simulink model "Sim_Ex32_Quiz"  (R2017a)
settings: Solver=VariableStepAuto  StartTime=0.0  StopTime=Stop_Time  MaxStep=100e-6  RelTol=1e-3
undefined symbols (not defined in the file or in its folder): Grid, PLL
settings Model: SimulationMode=accelerator  Creator=Joonhee  LastModifiedBy=Joonhee

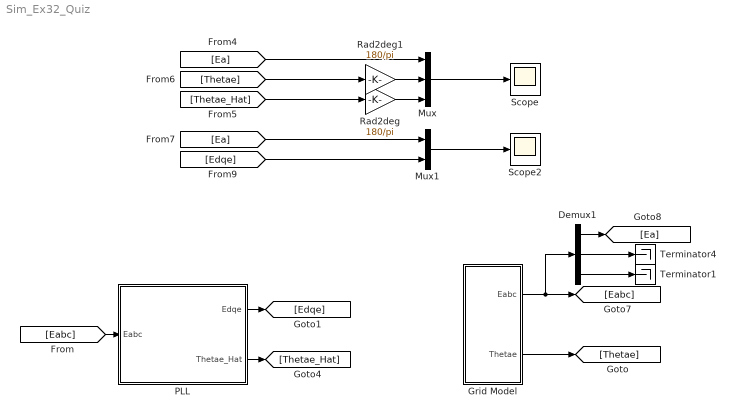
== system Sim_Ex32_Quiz ==
  Demux1 : Demux  Outputs=3
  Grid Model : Subsystem
  Mux : Mux  Inputs=3
  Mux1 : Mux  Inputs=2
  PLL : Subsystem  TreatAsAtomicUnit=on
  Rad2deg : Gain  Gain=180/pi
  Rad2deg1 : Gain  Gain=180/pi
  Scope : Scope
  Scope2 : Scope
  Terminator1 : Terminator
  Terminator4 : Terminator
  wires:
  Mux/1 -> Scope/1
  [Thetae_Hat] -> Rad2deg/1
  Rad2deg/1 -> Mux/3
  [Thetae] -> Rad2deg1/1
  Rad2deg1/1 -> Mux/2
  [Ea] -> Mux/1
  Mux1/1 -> Scope2/1
  [Ea] -> Mux1/1
  [Edqe] -> Mux1/2
  PLL/2(Thetae_Hat) -> [Thetae_Hat]
  PLL/1(Edqe) -> [Edqe]
  Demux1/1 -> [Ea]
  Demux1/2 -> Terminator4/1
  Demux1/3 -> Terminator1/1
  Grid Model/1(Eabc) -> Demux1/1, [Eabc]
  Grid Model/2(Thetae) -> [Thetae]
  [Eabc] -> PLL/1(Eabc)

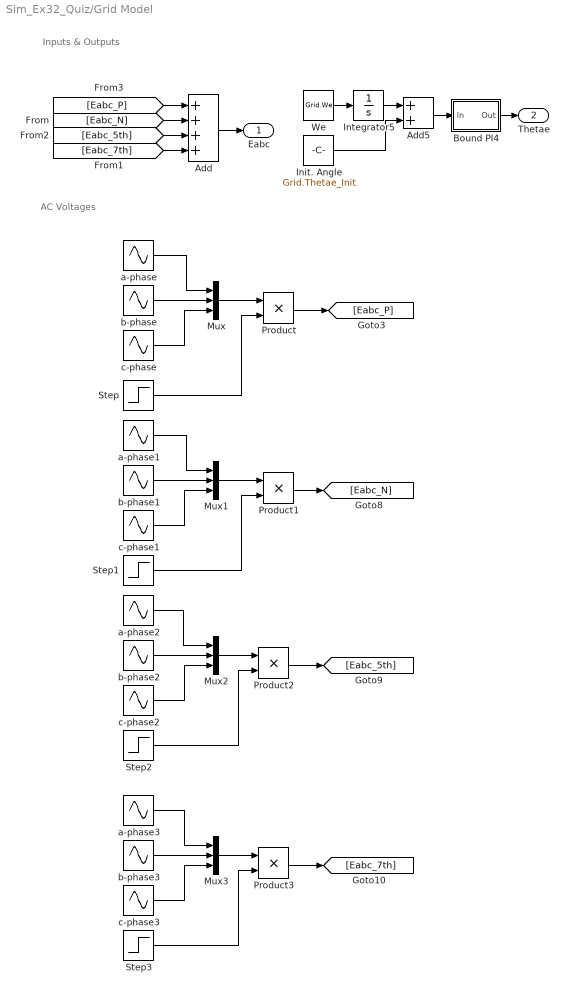
== system Sim_Ex32_Quiz/Grid Model ==
  note: AC Voltages
  note: Inputs & Outputs
  Add : Sum  Inputs=++++
  Add5 : Sum
  Bound PI4 : Subsystem
  Init. Angle : Constant  Value=Grid.Thetae_Init
  Integrator5 : Integrator
  Mux{,1..3} (4 alike) : Mux  Inputs=3
  Product{,1..3} (4 alike) : Product
  Step : Step  Time=Grid.Time_Fault  Before=1  After=Grid.Ratio_P  SampleTime=0
  Step1 : Step  Time=Grid.Time_Fault  SampleTime=0
  Step2 : Step  Time=Grid.Time_Fault  SampleTime=0
  Step3 : Step  Time=Grid.Time_Fault  SampleTime=0
  We : Constant  Value=Grid.We
  a-phase : Sin  Amplitude=Grid.V_P  Frequency=Grid.We  Phase=Grid.Thetae_Init+pi  SampleTime=0
  a-phase1 : Sin  Amplitude=Grid.V_N  Frequency=Grid.We  Phase=Grid.Thetae_N_Init+pi  SampleTime=0
  a-phase2 : Sin  Amplitude=Grid.V_5th  Frequency=5*Grid.We  Phase=Grid.Thetae_5th_Init+pi  SampleTime=0
  a-phase3 : Sin  Amplitude=Grid.V_7th  Frequency=7*Grid.We  Phase=Grid.Thetae_7th_Init+pi  SampleTime=0
  b-phase : Sin  Amplitude=Grid.V_P  Frequency=Grid.We  Phase=Grid.Thetae_Init+pi-2/3*pi  SampleTime=0
  b-phase1 : Sin  Amplitude=Grid.V_N  Frequency=Grid.We  Phase=Grid.Thetae_N_Init+pi+2/3*pi  SampleTime=0
  b-phase2 : Sin  Amplitude=Grid.V_5th  Frequency=5*Grid.We  Phase=Grid.Thetae_5th_Init+pi+2/3*pi  SampleTime=0
  b-phase3 : Sin  Amplitude=Grid.V_7th  Frequency=7*Grid.We  Phase=Grid.Thetae_7th_Init+pi-2/3*pi  SampleTime=0
  c-phase : Sin  Amplitude=Grid.V_P  Frequency=Grid.We  Phase=Grid.Thetae_Init+pi-4/3*pi  SampleTime=0
  c-phase1 : Sin  Amplitude=Grid.V_N  Frequency=Grid.We  Phase=Grid.Thetae_N_Init+pi+4/3*pi  SampleTime=0
  c-phase2 : Sin  Amplitude=Grid.V_5th  Frequency=5*Grid.We  Phase=Grid.Thetae_5th_Init+pi+4/3*pi  SampleTime=0
  c-phase3 : Sin  Amplitude=Grid.V_7th  Frequency=7*Grid.We  Phase=Grid.Thetae_7th_Init+pi-4/3*pi  SampleTime=0
  Eabc : Outport
  Thetae : Outport  Port=2
  wires:
  [Eabc_P] -> Add/1
  Add/1 -> Eabc/1
  [Eabc_N] -> Add/2
  [Eabc_5th] -> Add/3
  [Eabc_7th] -> Add/4
  Bound PI4/1(Out) -> Thetae/1
  Add5/1 -> Bound PI4/1(In)
  We/1 -> Integrator5/1
  Init. Angle/1 -> Add5/2
  Integrator5/1 -> Add5/1
  b-phase/1 -> Mux/2
  a-phase/1 -> Mux/1
  c-phase/1 -> Mux/3
  c-phase1/1 -> Mux1/3
  a-phase1/1 -> Mux1/1
  b-phase1/1 -> Mux1/2
  b-phase2/1 -> Mux2/2
  a-phase2/1 -> Mux2/1
  c-phase2/1 -> Mux2/3
  c-phase3/1 -> Mux3/3
  a-phase3/1 -> Mux3/1
  b-phase3/1 -> Mux3/2
  Mux/1 -> Product/1
  Mux1/1 -> Product1/1
  Step/1 -> Product/2
  Product/1 -> [Eabc_P]
  Step1/1 -> Product1/2
  Mux2/1 -> Product2/1
  Mux3/1 -> Product3/1
  Step2/1 -> Product2/2
  Step3/1 -> Product3/2
  Product1/1 -> [Eabc_N]
  Product2/1 -> [Eabc_5th]
  Product3/1 -> [Eabc_7th]

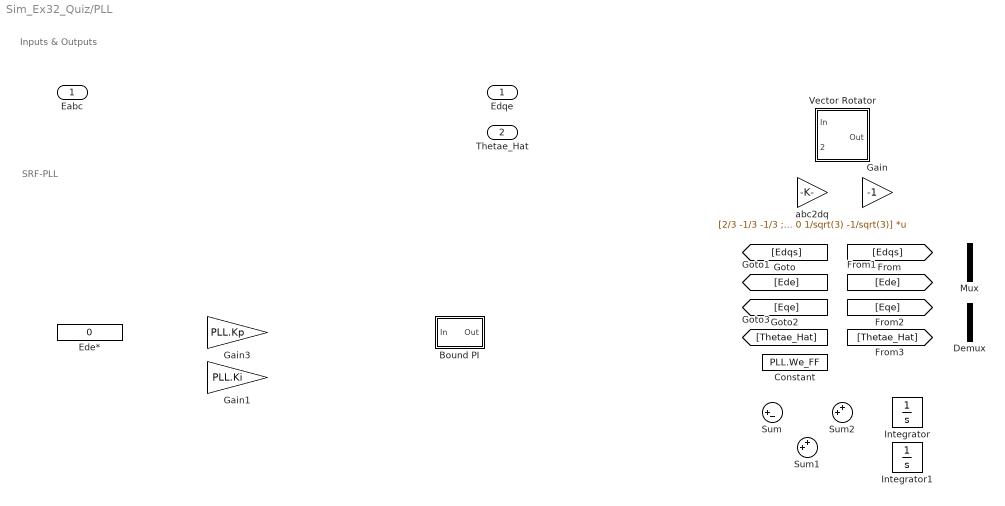
== system Sim_Ex32_Quiz/PLL ==
  note: Inputs & Outputs
  note: SRF-PLL
  Eabc : Inport
  Bound PI : Subsystem
  Constant : Constant  Value=PLL.We_FF
  Demux : Demux  Outputs=2
  Ede* : Constant  Value=0
  Gain : Gain  Gain=-1
  Gain1 : Gain  Gain=PLL.Ki
  Gain3 : Gain  Gain=PLL.Kp
  Integrator : Integrator
  Integrator1 : Integrator
  Mux : Mux  Inputs=2
  Sum : Sum  Inputs=|+-
  Sum1 : Sum  Inputs=++|
  Sum2 : Sum  Inputs=++|
  Vector Rotator : Subsystem  Tag=dqs2dqw
  abc2dq : Gain  Gain=[2/3 -1/3 -1/3 ; 0 1/sqrt(3) -1/sqrt(3)]  Multiplication=Matrix(K*u)  SaturateOnIntegerOverflow=on  OutDataTypeStr=Inherit: Same as input  ParamDataTypeStr=Inherit: Same as input
  Edqe : Outport
  Thetae_Hat : Outport  Port=2

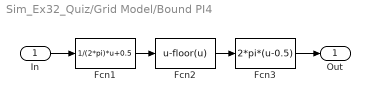
== system Sim_Ex32_Quiz/Grid Model/Bound PI4 ==
  In : Inport
  Fcn1 : Fcn  Expr=1/(2*pi)*u+0.5
  Fcn2 : Fcn  Expr=u-floor(u)
  Fcn3 : Fcn  Expr=2*pi*(u-0.5)
  Out : Outport
  wires:
  Fcn1/1 -> Fcn2/1
  Fcn2/1 -> Fcn3/1
  In/1 -> Fcn1/1
  Fcn3/1 -> Out/1

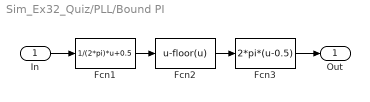
== system Sim_Ex32_Quiz/PLL/Bound PI ==
  In : Inport
  Fcn1 : Fcn  Expr=1/(2*pi)*u+0.5
  Fcn2 : Fcn  Expr=u-floor(u)
  Fcn3 : Fcn  Expr=2*pi*(u-0.5)
  Out : Outport
  wires:
  Fcn1/1 -> Fcn2/1
  Fcn2/1 -> Fcn3/1
  In/1 -> Fcn1/1
  Fcn3/1 -> Out/1

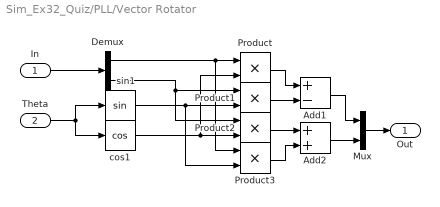
== system Sim_Ex32_Quiz/PLL/Vector Rotator ==
  In : Inport
  Theta : Inport  Port=2
  Add1 : Sum  Inputs=+-
  Add2 : Sum
  Demux : Demux  Outputs=2
  Mux : Mux  Inputs=[1 1]
  Product{,1..3} (4 alike) : Product  RndMeth=Zero
  cos1 : Trigonometry  Operator=cos
  sin1 : Trigonometry
  Out : Outport
  wires:
  Theta/1 -> cos1/1, sin1/1
  Demux/1 -> Product3/1, Product/1
  Mux/1 -> Out/1
  In/1 -> Demux/1
  Demux/2 -> Product1/1, Product2/1
  cos1/1 -> Product/2, Product2/2
  sin1/1 -> Product1/2, Product3/2
  Product/1 -> Add1/1
  Product1/1 -> Add1/2
  Add1/1 -> Mux/1
  Product2/1 -> Add2/1
  Product3/1 -> Add2/2
  Add2/1 -> Mux/2
